simulink model "GroupWork_ValerieLovesBuckConverter_Controller2"  (R2021b)
settings: Solver=FixedStepDiscrete  StartTime=0.0  StopTime=0.25  RelTol=1e-3
PreLoadFcn:
  | %
  | Fc=3780;                          % PWM Carrier frequency (Hz)
  | Ts_Power=1/Fc/200;         % Simscape Power Systems sample time (s)
  | Ts_Control=20*Ts_Power;  % Inverter Control system sample time (s)
InitFcn:
  | %
  | Fc=3780;                          % PWM Carrier frequency (Hz)
  | Ts_Power=1/Fc/200;         % Simscape Power Systems sample time (s)
  | Ts_Control=20*Ts_Power;  % Inverter Control system sample time (s)
undefined symbols (not defined in the file): Ion, Lithium
libraries: spsSeriesRLCBranchLib x5, spsDiodeLib x4, spsMosfetLib x2, spsPWMGeneratorDCDCLib x2, spsStairGeneratorLib x2, spsPVArrayLib x2, spsBatteryLib x1, spsCurrentMeasurementLib x1, spsVoltageMeasurementLib x1, spspowerguiLib x1
Description:
  | Copyright 2008-2019 The MathWorks, Inc.
settings Model: Creator=MathWorks  LastModifiedBy=ray
settings SolverCC: AlgebraicLoopSolver=TrustRegion
settings DataIOCC: SaveFormat=Structure  SignalLoggingSaveFormat=ModelDataLogs  SaveOutput=off  SignalLogging=off  DSMLogging=off  SaveTime=off  ReturnWorkspaceOutputs=off
settings OptimizationCC: ExpressionDepthLimit=2147483647  LifeSpan=inf
settings DebuggingCC: UnderspecifiedInitializationDetection=Classic  MergeDetectMultiDrivingBlocksExec=none  SolverPrmCheckMsg=warning  FcnCallInpInsideContextMsg=warning  AllowSymbolicDim=off  StateNameClashWarn=warning  SFUnexpectedBacktrackingDiag=warning  SFNoUnconditionalDefaultTransitionDiag=warning  SFExecutionAtInitializationDiag=none  SFMachineParentedDataDiag=warning  ArithmeticOperatorsInVariantConditions=warning
settings HardwareCC: ProdBitPerPointer=32  ProdBitPerSizeT=32  ProdBitPerPtrDiffT=32  ProdLargestAtomicFloat=None  ProdIntDivRoundTo=Undefined  ProdEndianess=Unspecified  ProdWordSize=32  ProdHWDeviceType=32-bit Generic
settings ModelReferenceCC: PropagateSignalLabelsOutOfModel=off
settings SFSimCC: SimUseLocalCustomCode=off  CustomCodeUndefinedFunction=UseInterfaceOnly
settings RTWCC: RTWUseLocalCustomCode=off
settings CodeAppCC: StateflowObjectComments=on
settings GRTTargetCC: TargetLangStandard=C89/C90 (ANSI)  CombineOutputUpdateFcns=off  GRTInterface=on
settings ConfigComp: CovMetricSettings=dw  CovSaveCumulativeToWorkspaceVar=on  CovSaveSingleToWorkspaceVar=on  CovExternalEMLEnable=off  CovSFcnEnable=off
settings SimscapeCC: SimscapeNormalizeSystem=off

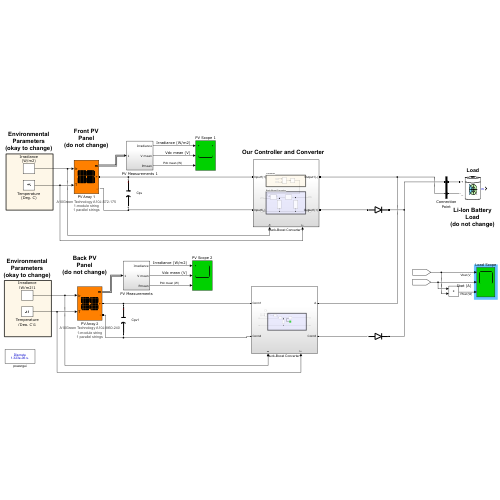
[thumbnail: Simulink's stored preview of the top-level diagram]
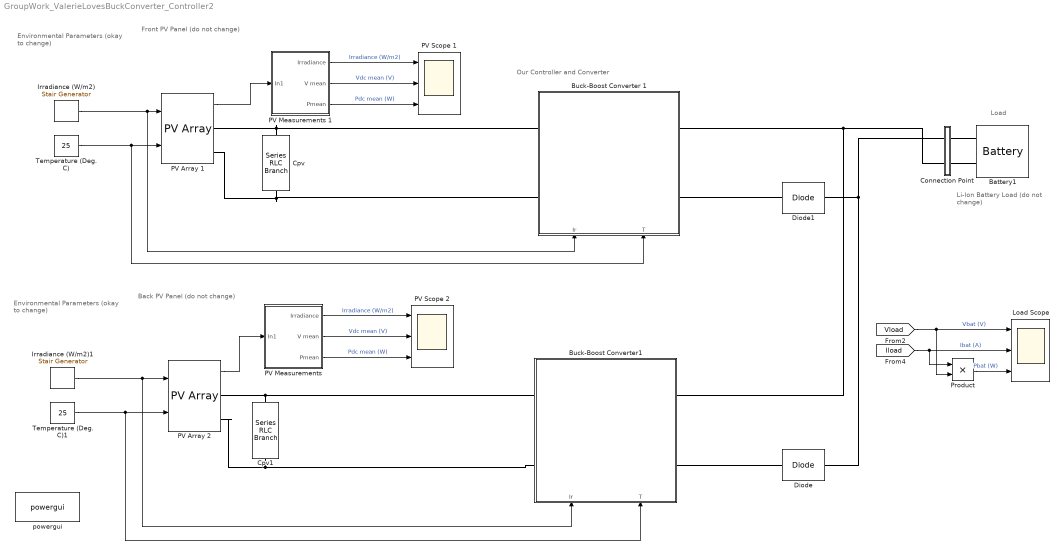
== system GroupWork_ValerieLovesBuckConverter_Controller2 ==
  note: Load
  note: Li-Ion Battery
      | Load
      | (do not change)
  note: Front PV
      | Panel
      | (do not change)
  note: Environmental
      | Parameters
      | (okay to change)
  note: Our Controller and Converter
  note: Environmental
      | Parameters
      | (okay to change)
  note: Back PV
      | Panel
      | (do not change)
  Battery1 : spsBatteryLib/Battery  BatType=Lithium-Ion  ShowTempParam=off  ThermalPreset=no  ShowAgeParam=off  NomV=100  NomQ=5  SOC=50  Batt_Tr=30  PresetModel=on  MaxQ=5  MinV=75  FullV=116.3987  Dis_rate=2.1739  R=0.2  Normal_OP=4.5217  expZone="[108.0386     0.2456522]"  current=[6.5 13 32.5]  Units=Time  Tci=20  NomT=20  T2=-30  MaxQ2=4.8  FullV2=7.1  Normal_OP2=5.655  expZone2="[6.58           1]"  Rca=0.6  ti=2000  Dp=0  Neq0=0  Tsim=1e6  Ta1=25  Qeol=5.4*0.9  Reol=0.013333*1.2  Char_age=[2.3478, 3]  Dis_age=[2.3478, 10]  N1=1500  N2=10500  N3=1000  N4=1400  Ta2=45  N5=950
  Buck-Boost Converter 1 : Subsystem
      settings: PortSchema="{\"entries\":[{\"content\":{\"sides\":[{\"content\":{\"connectorIds\":[\"LConn1\",\"LConn2\"]},\"type\":\"ConnectorPlacement.EquallySpacedRectSide\",\"uuid\":\"71107f47-ce51-452e-9179-51f8038779c5\"},{\"content\":{\"connectorIds\":[\"RConn1\",\"RConn2\"],\"side\":\"RIGHT\"},\"type\":\"ConnectorPlacement.EquallySpacedRectSide\",\"uuid\":\"312b1ac5-e0b8-4246-b858-aa3db1d4ff4c\"},{\"content\":{\"connectorIds\":[],\"side\":\"TOP\"},\"type\":\"ConnectorPlacement.EquallySpacedRectSide\",\"uuid\":\"8c8898a7-a002-46b7-a2c8-03b4ad08cbf3\"},{\"content\":{\"connectorIds\":[\"In1\",\"In2\"],\"side\":\"BOTTOM\"},\"type\":\"ConnectorPlacement.EquallySpacedRectSide\",\"uuid\":\"1ca7f4c2-2f50-459b-a853-5ac63f9172ad\"}]},\"type\":\"ConnectorPlacement.EquallySpacedConnector\",\"uuid\":\"275fbfe1-215d-4a27-8fa0-e68a8c379b2e\"}],\"packageUris\":[\"http://schema.mathworks.com/mf0/Connector/R2020b\"],\"version\":\"1.0\"}"
  Buck-Boost Converter1 : Subsystem
      settings: PortSchema="{\"entries\":[{\"content\":{\"sides\":[{\"content\":{\"connectorIds\":[\"LConn1\",\"LConn2\"]},\"type\":\"ConnectorPlacement.EquallySpacedRectSide\",\"uuid\":\"540095d8-fdf3-43c7-978a-c607389d9a56\"},{\"content\":{\"connectorIds\":[\"RConn1\",\"RConn2\"],\"side\":\"RIGHT\"},\"type\":\"ConnectorPlacement.EquallySpacedRectSide\",\"uuid\":\"db44d909-0859-415e-83df-7d00ca326b34\"},{\"content\":{\"connectorIds\":[],\"side\":\"TOP\"},\"type\":\"ConnectorPlacement.EquallySpacedRectSide\",\"uuid\":\"bd69e050-bdd9-458a-85b4-279e0eb927fb\"},{\"content\":{\"connectorIds\":[\"In1\",\"In2\"],\"side\":\"BOTTOM\"},\"type\":\"ConnectorPlacement.EquallySpacedRectSide\",\"uuid\":\"f55d3025-c291-44c0-b689-5c68fd8a2222\"}]},\"type\":\"ConnectorPlacement.EquallySpacedConnector\",\"uuid\":\"cfdd2a1b-3f9d-485a-a40f-262a49177e9a\"}],\"packageUris\":[\"http://schema.mathworks.com/mf0/Connector/R2020b\"],\"version\":\"1.0\"}"
  Connection Point : Subsystem
  Cpv : spsSeriesRLCBranchLib/Series RLC Branch  LConnTagsString=__new0  RConnTagsString=__new0  BranchType=C  Resistance=1  Inductance=1e-3  SetiL0=off  InitialCurrent=0  Capacitance=1e-5  Setx0=on  InitialVoltage=36  Measurements=None
  Cpv1 : spsSeriesRLCBranchLib/Series RLC Branch  LConnTagsString=__new0  RConnTagsString=__new0  BranchType=C  Resistance=1  Inductance=1e-3  SetiL0=off  InitialCurrent=0  Capacitance=1e-5  Setx0=on  InitialVoltage=36  Measurements=None
  Diode : spsDiodeLib/Diode  Ron=0.000001  Lon=0  Vf=0  IC=0  UseSnubber=0  Rs=0  Cs=0  Measurements=off
  Diode1 : spsDiodeLib/Diode  Ron=0.000001  Lon=0  Vf=0  IC=0  UseSnubber=0  Rs=0  Cs=0  Measurements=off
  Irradiance (W/m2) : spsStairGeneratorLib/Stair Generator  t=0  e=1000  Ts=Ts_Power
  Irradiance (W/m2)1 : spsStairGeneratorLib/Stair Generator  t=0  e=1000  Ts=Ts_Power
  Load Scope : Scope  NumInputPorts=3
  PV Array 1 : spsPVArrayLib/PV Array  Npar=1  Nser=1  PlotType=array @ 1000 W/m2 & specified temperatures  S_vec="[ 1000  500  100 ]"  Temp_C_vec=[ 45 25 100 ]  ModuleName=A10Green Technology A10J-S72-175  PlotWhenSelected=off  Pm=175.0914  Ncell=72  Voc=43.99  Isc=5.17  Vm=36.63  Im=4.78  beta_Voc_pc=-0.3616  alpha_Isc_pc=0.041509  beta_Voc=-0.15907  alpha_Isc=0.002146  IL=5.178  I0=1.7842e-10  nI=0.98852  Rsh=249.6758  Rs=0.38412  RobustModel=off  RobustCellTemperature=313.3991  BAL=on  Tc=1e-6  Tfilter=5e-5
      settings: AttributesFormatString=|
      | %<ModuleName>
      | %<Nser>-module string
      | %<Npar> parallel strings
  PV Array 2 : spsPVArrayLib/PV Array  Npar=1  Nser=1  PlotType=array @ 1000 W/m2 & specified temperatures  S_vec="[ 1000  500  100 ]"  Temp_C_vec=[ 45 25 100 ]  ModuleName=A10Green Technology A10J-M60-240  PlotWhenSelected=off  Pm=240.5376  Ncell=60  Voc=36.84  Isc=8.32  Vm=30.72  Im=7.83  beta_Voc_pc=-0.359  alpha_Isc_pc=0.096995  beta_Voc=-0.13226  alpha_Isc=0.00807  IL=8.3299  I0=2.8736e-10  nI=0.99259  Rsh=330.6558  Rs=0.19366  RobustModel=off  RobustCellTemperature=313.3991  BAL=on  Tc=1e-6  Tfilter=5e-5
      settings: AttributesFormatString=|
      | %<ModuleName>
      | %<Nser>-module string
      | %<Npar> parallel strings
  PV Measurements : Subsystem
  PV Measurements 1 : Subsystem
  PV Scope 1 : Scope  NumInputPorts=3
  PV Scope 2 : Scope  NumInputPorts=3
  Product : Product
  Temperature (Deg. C) : Constant  Value=25
  Temperature (Deg. C)1 : Constant  Value=25
  powergui : spspowerguiLib/powergui  Priority=1  SimulationMode=Discrete  SampleTime=Ts_Power  frequency=60  Iterations=50  frequencyindice=0  Pbase=100e6  ErrMax=1e-4  UnitsV=kV  UnitsW=MW  buscounter=0  FunctionMessages=off  echomessages=off  EnableUseOfTLC=off  CurrentSourceSwitches=off  DisableSnubberDevices=off  DisableRonSwitches=off  DisableVfSwitches=off  DisplayEquations=off  AutomaticDiscreteSolvers=off  SolverType=Tustin/Backward Euler (TBE)  Interpol=off  ExternalGateDelay=off  methode=off  Ts=0  x0status=blocks  SPID=off  SwTol=0  HookPort=off  NonlinearTolerance=0  nMaxIteration=15  ContinueOnMaxIteration=off  RestoreLinks=warning  ResistiveCurrentMeasurement=off  Frange=[0:2:500]  Ylog=off  Xlog=on  ShowGrid=off  save=off  variable=ZData  structure=VIgrid  ZoomFFT=off  StartTime=0.55  cycles=1  DisplayStyle=1  fundamental=60  FreqAxis=on  MaxFrequency=10000  frequencyindicesteady=1  RmsSteady=1  display=off
  wires:
  [Iload] -> Product/1, Load Scope/2  "Ibat (A)"
  Irradiance (W/m2)/1 -> PV Array 1/1, Buck-Boost Converter 1/1(Ir)
  Temperature (Deg. C)/1 -> PV Array 1/2, Buck-Boost Converter 1/2(T)
  PV Array 1/1 -> PV Measurements 1/1(In1)
  PV Measurements/2(V mean) -> PV Scope 2/2  "Vdc mean (V)"
  PV Measurements/1(Irradiance) -> PV Scope 2/1  "Irradiance (W/m2)"
  [Vload] -> Product/2, Load Scope/1  "Vbat (V)"
  Product/1 -> Load Scope/3  "Pbat (W)"
  PV Measurements/3(Pmean) -> PV Scope 2/3  "Pdc mean (W)"
  Temperature (Deg. C)1/1 -> PV Array 2/2, Buck-Boost Converter1/2(T)
  Irradiance (W/m2)1/1 -> PV Array 2/1, Buck-Boost Converter1/1(Ir)
  PV Measurements 1/1(Irradiance) -> PV Scope 1/1  "Irradiance (W/m2)"
  PV Measurements 1/3(Pmean) -> PV Scope 1/3  "Pdc mean (W)"
  PV Measurements 1/2(V mean) -> PV Scope 1/2  "Vdc mean (V)"
  PV Array 2/1 -> PV Measurements/1(In1)
  connections:
  Connection Point/RConn1 -- Battery1/LConn1
  Connection Point/RConn2 -- Battery1/LConn2
  Cpv/LConn1 -- Buck-Boost Converter 1/LConn1 -- PV Array 1/RConn1
  Cpv/RConn1 -- PV Array 1/RConn2 -- Buck-Boost Converter 1/LConn2
  Buck-Boost Converter1/LConn1 -- PV Array 2/RConn1 -- Cpv1/LConn1
  Cpv1/RConn1 -- PV Array 2/RConn2 -- Buck-Boost Converter1/LConn2
  Buck-Boost Converter1/RConn1 -- Connection Point/LConn2 -- Buck-Boost Converter 1/RConn1
  Diode1/LConn1 -- Buck-Boost Converter 1/RConn2
  Diode/LConn1 -- Buck-Boost Converter1/RConn2
  Diode/RConn1 -- Diode1/RConn1 -- Connection Point/LConn1

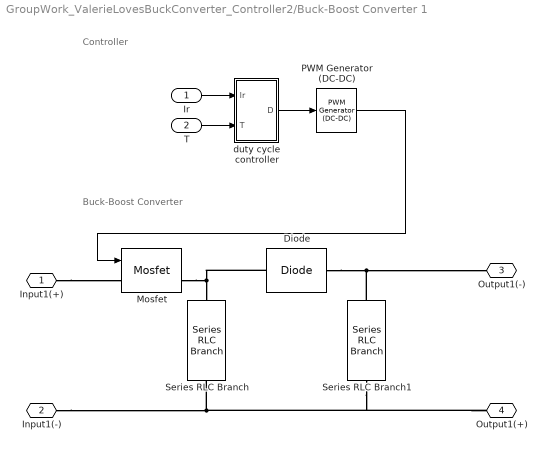
== system GroupWork_ValerieLovesBuckConverter_Controller2/Buck-Boost Converter 1 ==
  note: Buck-Boost Converter
  note: Controller
  Ir : Inport
  T : Inport  Port=2
  Diode : spsDiodeLib/Diode  Ron=0.001  Lon=0  Vf=0.8  IC=0  UseSnubber=0  Rs=500  Cs=250e-9  Measurements=off
  Mosfet : spsMosfetLib/Mosfet  Ron=0.1  Lon=0  Rd=0.01  Vfd=0  IC=0  Rs=1e5  Cs=inf  Measurements=on
  PWM Generator (DC-DC) : spsPWMGeneratorDCDCLib/PWM Generator (DC-DC)  Fsw=50000  Ts=0
  Series RLC Branch : spsSeriesRLCBranchLib/Series RLC Branch  LConnTagsString=__new0  RConnTagsString=__new0  BranchType=L  Resistance=1  Inductance=1e-3  SetiL0=off  InitialCurrent=0  Capacitance=1e-6  Setx0=off  InitialVoltage=0  Measurements=None
  Series RLC Branch1 : spsSeriesRLCBranchLib/Series RLC Branch  LConnTagsString=__new0  RConnTagsString=__new0  BranchType=C  Resistance=1  Inductance=1e-3  SetiL0=off  InitialCurrent=0  Capacitance=5e-12  Setx0=off  InitialVoltage=0  Measurements=None
  duty cycle controller : Subsystem
  Input1(+) : PMIOPort  Side=Left
  Input1(-) : PMIOPort  Port=2  Side=Left
  Output1(-) : PMIOPort  Port=3  Side=Right
  Output1(+) : PMIOPort  Port=4  Side=Right
  wires:
  PWM Generator (DC-DC)/1 -> Mosfet/1
  T/1 -> duty cycle controller/2(T)
  Ir/1 -> duty cycle controller/1(lr)
  duty cycle controller/1(D) -> PWM Generator (DC-DC)/1
  connections:
  Diode/LConn1 -- Output1(-)/RConn1 -- Series RLC Branch1/RConn1
  Mosfet/RConn1 -- Series RLC Branch/LConn1 -- Diode/RConn1
  Input1(+)/RConn1 -- Mosfet/LConn1
  Output1(+)/RConn1 -- Series RLC Branch1/LConn1 -- Input1(-)/RConn1 -- Series RLC Branch/RConn1

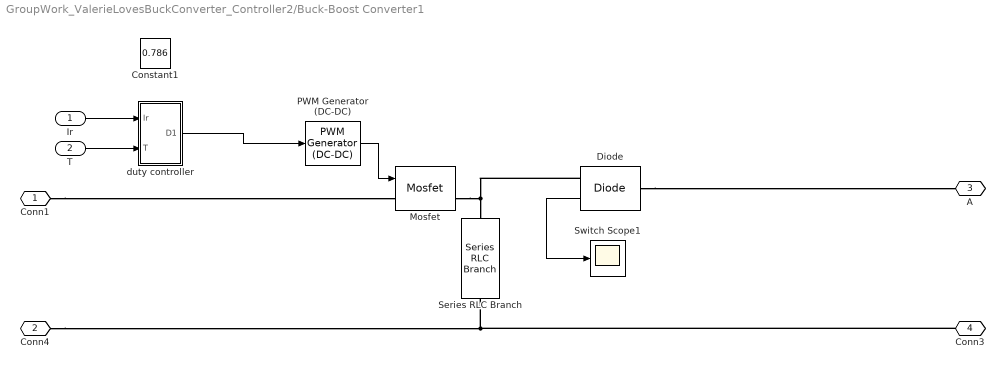
== system GroupWork_ValerieLovesBuckConverter_Controller2/Buck-Boost Converter1 ==
  Ir : Inport
  T : Inport  Port=2
  Constant1 : Constant  Value=0.786
  Diode : spsDiodeLib/Diode  Ron=0.001  Lon=0  Vf=0.8  IC=0  UseSnubber=0  Rs=500  Cs=250e-9  Measurements=on
  Mosfet : spsMosfetLib/Mosfet  Ron=0.1  Lon=0  Rd=0.01  Vfd=0  IC=0  Rs=1e5  Cs=inf  Measurements=on
  PWM Generator (DC-DC) : spsPWMGeneratorDCDCLib/PWM Generator (DC-DC)  Fsw=50000  Ts=0
  Series RLC Branch : spsSeriesRLCBranchLib/Series RLC Branch  LConnTagsString=__new0  RConnTagsString=__new0  BranchType=L  Resistance=1  Inductance=1e-3  SetiL0=off  InitialCurrent=0  Capacitance=1e-6  Setx0=off  InitialVoltage=0  Measurements=None
  Switch Scope1 : Scope
  duty controller : Subsystem
  Conn1 : PMIOPort  Side=Left
  Conn4 : PMIOPort  Port=2  Side=Left
  A : PMIOPort  Port=3  Side=Right
  Conn3 : PMIOPort  Port=4  Side=Right
  wires:
  Diode/1 -> Switch Scope1/1
  PWM Generator (DC-DC)/1 -> Mosfet/1
  Ir/1 -> duty controller/1(lr)
  T/1 -> duty controller/2(T)
  duty controller/1(D1) -> PWM Generator (DC-DC)/1
  connections:
  Diode/LConn1 -- A/RConn1
  Mosfet/RConn1 -- Series RLC Branch/LConn1 -- Diode/RConn1
  Conn1/RConn1 -- Mosfet/LConn1
  Conn3/RConn1 -- Conn4/RConn1 -- Series RLC Branch/RConn1

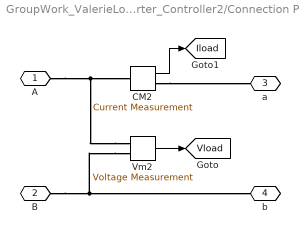
== system GroupWork_ValerieLovesBuckConverter_Controller2/Connection Point ==
  CM2 : spsCurrentMeasurementLib/Current Measurement  PhasorSimulation=off  OutputType=Complex  PSBequivalent=0
  Vm2 : spsVoltageMeasurementLib/Voltage Measurement  PhasorSimulation=off  OutputType=Complex  PSBequivalent=0
  A : PMIOPort  Side=Left
  B : PMIOPort  Port=2  Side=Left
  a : PMIOPort  Port=3  Side=Right
  b : PMIOPort  Port=4  Side=Right
  tag scope: Iload=global, Vload=global
  wires:
  Vm2/1 -> [Vload]
  CM2/1 -> [Iload]
  connections:
  Vm2/LConn2 -- b/RConn1 -- B/RConn1
  Vm2/LConn1 -- A/RConn1 -- CM2/LConn1
  CM2/RConn1 -- a/RConn1

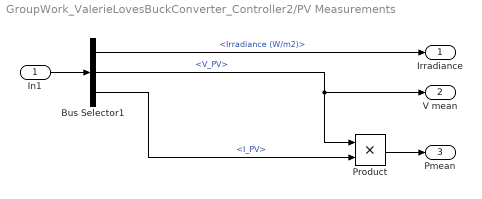
== system GroupWork_ValerieLovesBuckConverter_Controller2/PV Measurements ==
  In1 : Inport
  Bus Selector1 : BusSelector  OutputSignals=Irradiance (W/m2),V_PV,I_PV
  Product : Product
  Irradiance : Outport  VectorParamsAs1DForOutWhenUnconnected=off
  V mean : Outport  Port=2  VectorParamsAs1DForOutWhenUnconnected=off
  Pmean : Outport  Port=3  VectorParamsAs1DForOutWhenUnconnected=off
  wires:
  In1/1 -> Bus Selector1/1
  Bus Selector1/2 -> Product/1, V mean/1  "<V_PV>"
  Bus Selector1/3 -> Product/2  "<I_PV>"
  Bus Selector1/1 -> Irradiance/1  "<Irradiance (W/m2)>"
  Product/1 -> Pmean/1

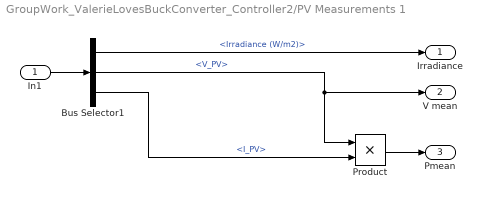
== system GroupWork_ValerieLovesBuckConverter_Controller2/PV Measurements 1 ==
  In1 : Inport
  Bus Selector1 : BusSelector  OutputSignals=Irradiance (W/m2),V_PV,I_PV
  Product : Product
  Irradiance : Outport  VectorParamsAs1DForOutWhenUnconnected=off
  V mean : Outport  Port=2  VectorParamsAs1DForOutWhenUnconnected=off
  Pmean : Outport  Port=3  VectorParamsAs1DForOutWhenUnconnected=off
  wires:
  In1/1 -> Bus Selector1/1
  Bus Selector1/2 -> Product/1, V mean/1  "<V_PV>"
  Bus Selector1/3 -> Product/2  "<I_PV>"
  Bus Selector1/1 -> Irradiance/1  "<Irradiance (W/m2)>"
  Product/1 -> Pmean/1

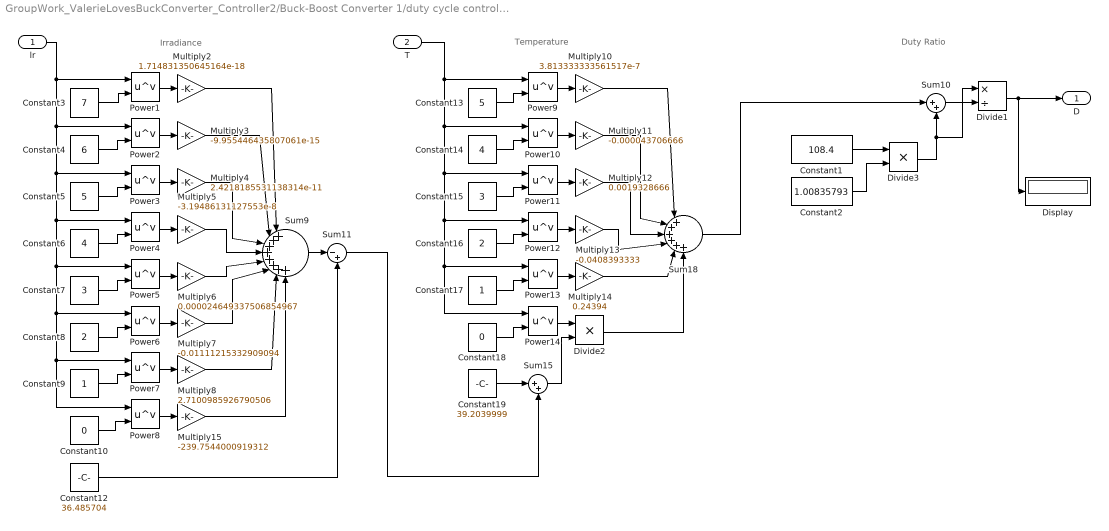
== system GroupWork_ValerieLovesBuckConverter_Controller2/Buck-Boost Converter 1/duty cycle controller ==
  note: Irradiance
  note: Temperature
  note: Duty Ratio
  lr : Inport
  T : Inport  Port=2
  Constant1 : Constant  Value=108.4
  Constant10 : Constant  Value=0
  Constant12 : Constant  Value=36.485704
  Constant13 : Constant  Value=5
  Constant14 : Constant  Value=4
  Constant15 : Constant  Value=3
  Constant16 : Constant  Value=2
  Constant17 : Constant
  Constant18 : Constant  Value=0
  Constant19 : Constant  Value=39.2039999
  Constant2 : Constant  Value=1.00835793
  Constant3 : Constant  Value=7
  Constant4 : Constant  Value=6
  Constant5 : Constant  Value=5
  Constant6 : Constant  Value=4
  Constant7 : Constant  Value=3
  Constant8 : Constant  Value=2
  Constant9 : Constant
  Display : Display
  Divide1 : Product  Inputs=*/
  Divide2 : Product  Inputs=**
  Divide3 : Product  Inputs=**
  Multiply10 : Gain  Gain=3.813333333561517e-7
  Multiply11 : Gain  Gain=-0.000043706666
  Multiply12 : Gain  Gain=0.0019328666
  Multiply13 : Gain  Gain=-0.0408393333
  Multiply14 : Gain  Gain=0.24394
  Multiply15 : Gain  Gain=-239.7544000919312
  Multiply2 : Gain  Gain=1.714831350645164e-18
  Multiply3 : Gain  Gain=-9.955446435807061e-15
  Multiply4 : Gain  Gain=2.4218185531138314e-11
  Multiply5 : Gain  Gain=-3.19486131127553e-8
  Multiply6 : Gain  Gain=0.000024649337506854967
  Multiply7 : Gain  Gain=-0.01111215332909094
  Multiply8 : Gain  Gain=2.7100985926790506
  Power{1..14} (14 alike) : Math  Operator=pow  SaturateOnIntegerOverflow=on
  Sum10 : Sum  Inputs=|++
  Sum11 : Sum  Inputs=|-+
  Sum15 : Sum  Inputs=|++
  Sum18 : Sum  Inputs=|++++++
  Sum9 : Sum  Inputs=|++++++++
  D : Outport
  wires:
  Constant16/1 -> Power12/2
  Power13/1 -> Multiply14/1
  Constant14/1 -> Power10/2
  Constant17/1 -> Power13/2
  Power10/1 -> Multiply11/1
  Power12/1 -> Multiply13/1
  Constant15/1 -> Power11/2
  Constant13/1 -> Power9/2
  Constant9/1 -> Power7/2
  Constant10/1 -> Power8/2
  Multiply6/1 -> Sum9/5
  Power2/1 -> Multiply3/1
  Multiply8/1 -> Sum9/7
  Constant8/1 -> Power6/2
  Power7/1 -> Multiply8/1
  Power9/1 -> Multiply10/1
  Constant7/1 -> Power5/2
  Constant4/1 -> Power2/2
  Sum10/1 -> Divide1/2
  Power11/1 -> Multiply12/1
  Multiply2/1 -> Sum9/1
  Power6/1 -> Multiply7/1
  Power5/1 -> Multiply6/1
  Constant18/1 -> Power14/2
  Constant6/1 -> Power4/2
  Constant3/1 -> Power1/2
  Constant12/1 -> Sum11/2
  Multiply4/1 -> Sum9/3
  Constant19/1 -> Sum15/1
  Power3/1 -> Multiply4/1
  Constant5/1 -> Power3/2
  Power4/1 -> Multiply5/1
  Divide3/1 -> Divide1/1, Sum10/2
  lr/1 -> Power2/1, Power3/1, Power4/1, Power5/1, Power8/1, Power7/1, Power6/1, Power1/1
  Power1/1 -> Multiply2/1
  Divide1/1 -> Display/1, D/1
  T/1 -> Power9/1, Power11/1, Power14/1, Power13/1, Power12/1, Power10/1
  Power8/1 -> Multiply15/1
  Sum9/1 -> Sum11/1
  Power14/1 -> Divide2/1
  Sum11/1 -> Sum15/2
  Sum15/1 -> Divide2/2
  Sum18/1 -> Sum10/1
  Constant1/1 -> Divide3/1
  Constant2/1 -> Divide3/2
  Multiply3/1 -> Sum9/2
  Multiply5/1 -> Sum9/4
  Multiply7/1 -> Sum9/6
  Multiply15/1 -> Sum9/8
  Multiply10/1 -> Sum18/1
  Multiply11/1 -> Sum18/2
  Multiply12/1 -> Sum18/3
  Multiply13/1 -> Sum18/4
  Multiply14/1 -> Sum18/5
  Divide2/1 -> Sum18/6

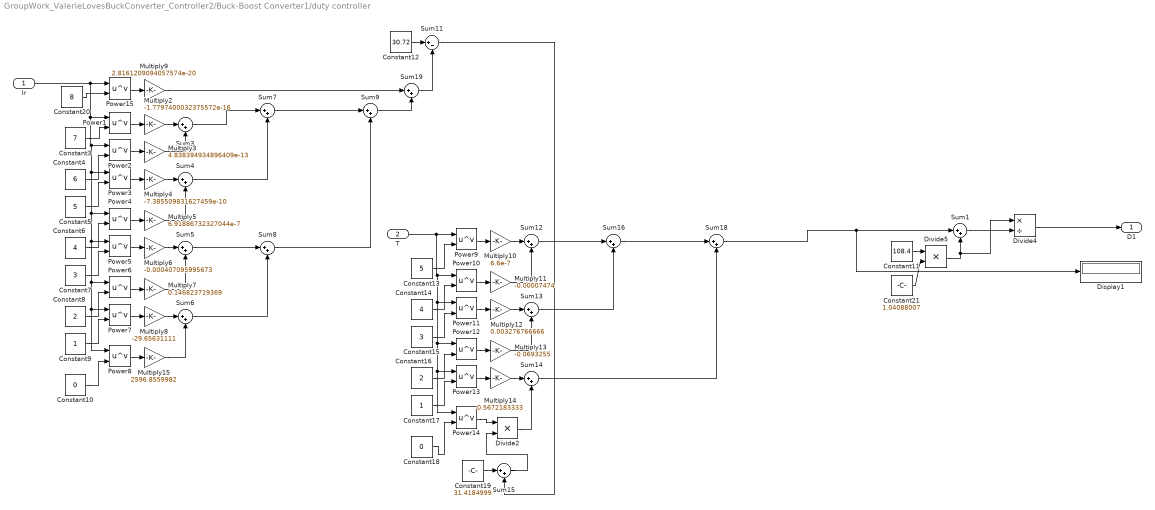
== system GroupWork_ValerieLovesBuckConverter_Controller2/Buck-Boost Converter1/duty controller ==
  lr : Inport
  T : Inport  Port=2
  Constant10 : Constant  Value=0
  Constant11 : Constant  Value=108.4
  Constant12 : Constant  Value=30.72
  Constant13 : Constant  Value=5
  Constant14 : Constant  Value=4
  Constant15 : Constant  Value=3
  Constant16 : Constant  Value=2
  Constant17 : Constant
  Constant18 : Constant  Value=0
  Constant19 : Constant  Value=31.4184999
  Constant20 : Constant  Value=8
  Constant21 : Constant  Value=1.04088007
  Constant3 : Constant  Value=7
  Constant4 : Constant  Value=6
  Constant5 : Constant  Value=5
  Constant6 : Constant  Value=4
  Constant7 : Constant  Value=3
  Constant8 : Constant  Value=2
  Constant9 : Constant
  Display1 : Display
  Divide2 : Product  Inputs=**
  Divide4 : Product  Inputs=*/
  Divide5 : Product  Inputs=**
  Multiply10 : Gain  Gain=6.6e-7
  Multiply11 : Gain  Gain=-0.00007474
  Multiply12 : Gain  Gain=0.003276766666
  Multiply13 : Gain  Gain=-0.0693255
  Multiply14 : Gain  Gain=0.5672183333
  Multiply15 : Gain  Gain=2596.8559982
  Multiply2 : Gain  Gain=-1.7797400032375572e-16
  Multiply3 : Gain  Gain=4.838394934896409e-13
  Multiply4 : Gain  Gain=-7.385509831627459e-10
  Multiply5 : Gain  Gain=6.91886732327044e-7
  Multiply6 : Gain  Gain=-0.000407095995673
  Multiply7 : Gain  Gain=0.146823719369
  Multiply8 : Gain  Gain=-29.65631111
  Multiply9 : Gain  Gain=2.8161209094057574e-20
  Power{1..15} (15 alike) : Math  Operator=pow  SaturateOnIntegerOverflow=on
  Sum{1,3..9,12..16,18..19} (15 alike) : Sum  Inputs=|++
  Sum11 : Sum  Inputs=|+-
  D1 : Outport
  wires:
  Sum9/1 -> Sum19/2
  Power15/1 -> Multiply9/1
  Multiply9/1 -> Sum19/1
  Constant16/1 -> Power12/2
  Power13/1 -> Multiply14/1
  Multiply10/1 -> Sum12/1
  Constant14/1 -> Power10/2
  Constant17/1 -> Power13/2
  Power10/1 -> Multiply11/1
  Multiply11/1 -> Sum12/2
  Sum16/1 -> Sum18/1
  Multiply14/1 -> Sum14/1
  Multiply12/1 -> Sum13/1
  Power12/1 -> Multiply13/1
  Constant15/1 -> Power11/2
  Sum12/1 -> Sum16/1
  Constant13/1 -> Power9/2
  Constant9/1 -> Power7/2
  Constant10/1 -> Power8/2
  Multiply3/1 -> Sum3/2
  Multiply6/1 -> Sum5/1
  Power2/1 -> Multiply3/1
  Multiply8/1 -> Sum6/1
  Constant20/1 -> Power15/2
  Constant8/1 -> Power6/2
  Sum7/1 -> Sum9/1
  Power7/1 -> Multiply8/1
  Power9/1 -> Multiply10/1
  Sum8/1 -> Sum9/2
  Constant7/1 -> Power5/2
  Constant4/1 -> Power2/2
  Power11/1 -> Multiply12/1
  Sum5/1 -> Sum8/1
  Multiply2/1 -> Sum3/1
  Multiply7/1 -> Sum5/2
  Power6/1 -> Multiply7/1
  Power5/1 -> Multiply6/1
  Multiply13/1 -> Sum13/2
  Constant18/1 -> Power14/2
  Sum6/1 -> Sum8/2
  Constant6/1 -> Power4/2
  Constant3/1 -> Power1/2
  Sum13/1 -> Sum16/2
  Sum3/1 -> Sum7/1
  Constant12/1 -> Sum11/1
  Multiply4/1 -> Sum4/1
  Constant19/1 -> Sum15/1
  Sum4/1 -> Sum7/2
  Power3/1 -> Multiply4/1
  Constant5/1 -> Power3/2
  Power4/1 -> Multiply5/1
  Multiply5/1 -> Sum4/2
  lr/1 -> Power15/1, Power5/1, Power8/1, Power7/1, Power6/1, Power4/1, Power3/1, Power2/1, Power1/1
  Sum15/1 -> Divide2/2
  Power1/1 -> Multiply2/1
  T/1 -> Power14/1, Power13/1, Power12/1, Power11/1, Power10/1, Power9/1
  Divide5/1 -> Divide4/1, Sum1/2
  Constant11/1 -> Divide5/1
  Constant21/1 -> Divide5/2
  Divide4/1 -> D1/1
  Sum1/1 -> Divide4/2
  Sum19/1 -> Sum11/2
  Power14/1 -> Divide2/1
  Power8/1 -> Multiply15/1
  Multiply15/1 -> Sum6/2
  Divide2/1 -> Sum14/2
  Sum11/1 -> Sum15/2
  Sum18/1 -> Display1/1, Sum1/1
  Sum14/1 -> Sum18/2
